simulink model "invers_dynamics_exo"  (R2023a)
settings: Solver=FixedStepAuto  StartTime=0.0  StopTime=20  RelTol=1e-3
libraries: simulink x6
settings Model: Creator=tobia  LastModifiedBy=tobia
settings OptimizationCC: OptimizeBlockIOStorage=off  ZeroExternalMemoryAtStartup=off  ZeroInternalMemoryAtStartup=off  OptimizeDataStoreBuffers=off  BusAssignmentInplaceUpdate=off
settings DebuggingCC: SFUnexpectedBacktrackingDiag=warning  SFNoUnconditionalDefaultTransitionDiag=warning
settings RTWCC: GenCodeOnly=on  GenerateReport=on  Toolchain=Microsoft Visual C++ 2022 v17.0 | CMake/nmake (64-bit Windows)  BuildConfiguration=Debug  LaunchReport=on  TargetLang=C++
settings CodeAppCC: ForceParamTrailComments=on  MATLABSourceComments=on  EnableCustomComments=on
settings GRTTargetCC: TargetLangStandard=C++11 (ISO)  CombineSignalStateStructs=on  CodeInterfacePackaging=C++ class  SupportVariableSizeSignals=on  MultiInstanceErrorCode=Warning

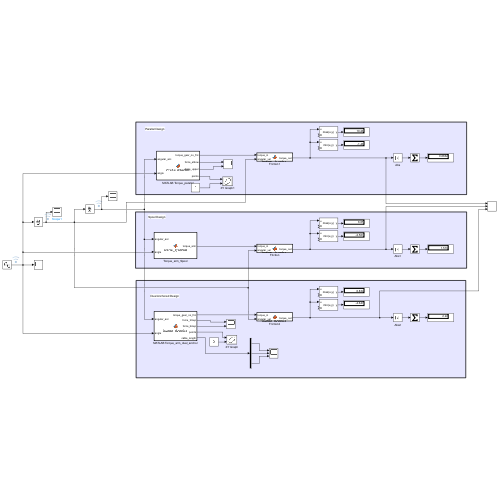
[thumbnail: Simulink's stored preview of the top-level diagram]
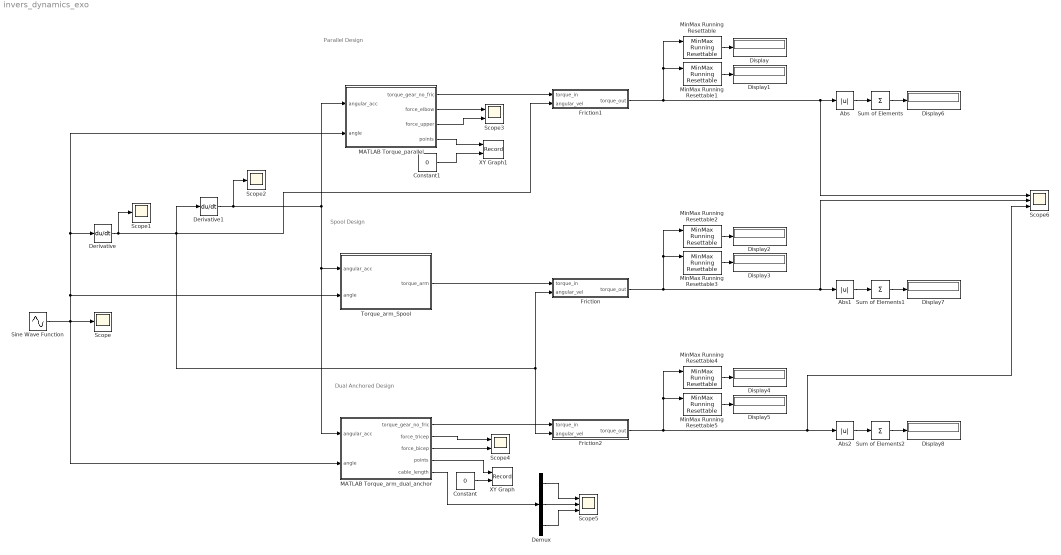
== system invers_dynamics_exo ==
  note: Dual Anchored Design
  note: Spool Design
  note: Parallel Design
  Abs : Abs  SaturateOnIntegerOverflow=off
  Abs1 : Abs  SaturateOnIntegerOverflow=off
  Abs2 : Abs  SaturateOnIntegerOverflow=off
  Constant : Constant  Value=0
  Constant1 : Constant  Value=0
  Demux : Demux  Outputs=3
  Derivative : Derivative
  Derivative1 : Derivative
  Display{,1..8} (9 alike) : Display
  Friction : MATLAB Function  TreatAsAtomicUnit=on
  Friction1 : MATLAB Function  TreatAsAtomicUnit=on
  Friction2 : MATLAB Function  TreatAsAtomicUnit=on
  MATLAB Torque_arm_dual_anchor : MATLAB Function  TreatAsAtomicUnit=on
  MATLAB Torque_parallel : MATLAB Function  TreatAsAtomicUnit=on
  MinMax Running Resettable : simulink/Math Operations/MinMax Running Resettable  Function=max  vinit=0.0
  MinMax Running Resettable1 : simulink/Math Operations/MinMax Running Resettable  Function=min  vinit=0.0
  MinMax Running Resettable2 : simulink/Math Operations/MinMax Running Resettable  Function=max  vinit=0.0
  MinMax Running Resettable3 : simulink/Math Operations/MinMax Running Resettable  Function=min  vinit=0.0
  MinMax Running Resettable4 : simulink/Math Operations/MinMax Running Resettable  Function=max  vinit=0.0
  MinMax Running Resettable5 : simulink/Math Operations/MinMax Running Resettable  Function=min  vinit=0.0
  Scope : Scope
  Scope1 : Scope
  Scope2 : Scope
  Scope3 : Scope  NumInputPorts=2
  Scope4 : Scope  NumInputPorts=2
  Scope5 : Scope  NumInputPorts=3
  Scope6 : Scope  NumInputPorts=3
  Sine Wave Function : Sin  Amplitude=57.5*pi/180  Bias=57.5*pi/180  Frequency=0.5  Phase=4  SampleTime=0.01
  Sum of Elements : Sum  Inputs=+
  Sum of Elements1 : Sum  Inputs=+
  Sum of Elements2 : Sum  Inputs=+
  Torque_arm_Spool : MATLAB Function  TreatAsAtomicUnit=on
  XY Graph : Record  FileSettingsInternal="{\"entries\":[{\"content\":{\"excelSettings\":{\"content\":{},\"type\":\"Streamout.ExcelSettings\"}},\"type\":\"Streamout.FileSettingStorage\",\"uuid\":\"90cafc74-587b-4871-8b77-8289e6956aa1\"}],\"packageUris\":[\"http://schema.mathworks.com/mf0/streamout_blocks/R2020a\"],\"version\":\"1.0\"}"  Layout=[1 1]  SignalsInternal="{\"entries\":[{\"content\":{\"signals\":[{\"content\":{\"blockPath\":[\"invers_dynamics_exo/XY Graph\"],\"dimensions\":[1,8],\"domain\":\"invers_dynamics_exo/XY Graph\",\"hasChildren\":true,\"lineColor\":\"#ff13a6\",\"port\":1,\"sid\":[\"\"],\"signalID\":426,\"signalName\":\"MATLAB Torque_arm_dual_anchor:4\"},\"type\":\"RecordBlkView.Signal\",\"uuid\":\"f57bbfb4-fc0c-47c9-ab87-1a3b218e2124\"},{\"content\":{\"blockPath\":[\"invers_dynamics_exo/XY Graph\"],\"channel\":[1,1],\"dimensions\":[1,8],\"domain\":\"invers_dynamics_exo/XY Graph\",\"lineColor\":\"#7e2f8e\",\"parentID\":426,\"plots\":[1],\"port\":1,\"sid\":[\"\"],\"signalID\":427,\"signalName\":\"MATLAB Torque_arm_dual_anchor:4\"},\"type\":\"RecordBlkView.Signal\",\"uuid\":\"17954e79-1570-4b7c-beb2-87390e5cb58c\"},{\"content\":{\"blockPath\":[\"invers_dynamics_exo/XY Graph\"],\"dimensions\":[1],\"domain\":\"invers_dynamics_exo/XY Graph\",\"lineColor\":\"#a2142f\",\"plots\":[1],\"port\":2,\"sid\":[\"\"],\"signalID\":436,\"signalName\":\"Constant\"},\"type\":\"RecordBlkView.Signal\",\"uuid\":\"88e606e6-8988-44ae-93fd-16471fbb4abb\"},{\"content\":{\"blockPath\":[\"invers_dynamics_exo/XY Graph\"],\"channel\":[1,2],\"dimensions\":[1,8],\"domain\":\"invers_dynamics_exo/XY Graph\",\"lineColor\":\"#64d413\",\"parentID\":426,\"plots\":[1],\"port\":1,\"sid\":[\"\"],\"signalID\":497,\"signalName\":\"MATLAB Torque_arm_dual_anchor:4\"},\"type\":\"RecordBlkView.Signal\",\"uuid\":\"809d9a61-5690-47a9-8092-efb78bb0c7b6\"},{\"content\":{\"blockPath\":[\"invers_dynamics_exo/XY Graph\"],\"channel\":[1,3],\"dimensions\":[1,8],\"domain\":\"invers_dynamics_exo/XY Graph\",\"lineColor\":\"#ff13a6\",\"parentID\":426,\"plots\":[1],\"port\":1,\"sid\":[\"\"],\"signalID\":498,\"signalName\":\"MATLAB Torque_arm_dual_anchor:4\"},\"type\":\"RecordBlkView.Signal\",\"uuid\":\"46f14f9b-1d62-4e7a-9e42-de28faff6f15\"},{\"content\":{\"blockPath\":[\"invers_dynamics_exo/XY Graph\"],\"channel\":[1,4],\"dimensions\":[1,8],\"domain\":\"invers_dynamics_exo/XY Graph\",\"lineColor\":\"#fe330a\",\"parentID\":426,\"plots\":[1],\"port\":1,\"sid\":[\"\"],\"signalID\":499,\"signalName\":\"MATLAB Torque_arm_dual_anchor:4\"},\"type\":\"RecordBlkView.Signal\",\"uuid\":\"354214a8-296c-4194-9ecc-28dd992aaaef\"},{\"content\":{\"blockPath\":[\"invers_dynamics_exo/XY Graph\"],\"channel\":[1,5],\"dimensions\":[1,8],\"domain\":\"invers_dynamics_exo/XY Graph\",\"lineColor\":\"#22b573\",\"parentID\":426,\"plots\":[1],\"port\":1,\"sid\":[\"\"],\"signalID\":500,\"signalName\":\"MATLAB Torque_arm_dual_anchor:4\"},\"type\":\"RecordBlkView.Signal\",\"uuid\":\"e2127789-c763-4787-91a7-13d7228fb6b6\"},{\"content\":{\"blockPath\":[\"invers_dynamics_exo/XY Graph\"],\"channel\":[1,6],\"dimensions\":[1,8],\"domain\":\"invers_dynamics_exo/XY Graph\",\"lineColor\":\"#0072bd\",\"parentID\":426,\"plots\":[1],\"port\":1,\"sid\":[\"\"],\"signalID\":501,\"signalName\":\"MATLAB Torque_arm_dual_anchor:4\"},\"type\":\"RecordBlkView.Signal\",\"uuid\":\"b365466d-55b6-410a-a4a0-64c454fc3450\"},{\"content\":{\"blockPath\":[\"invers_dynamics_exo/XY Graph\"],\"channel\":[1,7],\"dimensions\":[1,8],\"domain\":\"invers_dynamics_exo/XY Graph\",\"lineColor\":\"#d95319\",\"parentID\":426,\"plots\":[1],\"port\":1,\"sid\":[\"\"],\"signalID\":502,\"signalName\":\"MATLAB Torque_arm_dual_anchor:4\"},\"type\":\"RecordBlkView.Signal\",\"uuid\":\"c2ca46fb-f305-425c-9fde-4563dfa5b76e\"},{\"content\":{\"blockPath\":[\"invers_dynamics_exo/XY Graph\"],\"channel\":[1,8],\"dimensions\":[1,8],\"domain\":\"invers_dynamics_exo/XY Graph\",\"lineColor\":\"#edb120\",\"parentID\":426,\"plots\":[1],\"port\":1,\"sid\":[\"\"],\"signalID\":503,\"signalName\":\"MATLAB Torque_arm_dual_anchor:4\"},\"type\":\"RecordBlkView.Signal\",\"uuid\":\"76ece406-2e19-4193-9589-b77808bf0ec4\"}]},\"type\":\"RecordBlkView.InputSignals\",\"uuid\":\"c80cf8b0-44b7-4c38-9eaf-bf62f72da6b7\"}],\"packageUris\":[\"http://schema.mathworks.com/mf0/streamout_blocks/R2020a\"],\"version\":\"1.0\"}"  VisualizationBindings="{\"xyplotplugin\":{\"info\":[{\"series\":[{\"bindingParametersList\":[{\"parameter\":\"X-Axis\",\"signalID\":498,\"signalName\":\"MATLAB Torque_arm_dual_anchor:4(1,3)\"},{\"parameter\":\"Y-Axis\",\"signalID\":499,\"signalName\":\"MATLAB Torque_arm_dual_anchor:4(1,4)\"}],\"seriesID\":23966},{\"bindingParametersList\":[{\"parameter\":\"X-Axis\",\"signalID\":436,\"signalName\":\"Constant\"},{\"parameter\":\"Y-Axis\",\"signalID\":436,\"signalName\":\"Constant\"}],\"seriesID\":54397},{\"bindingParametersList\":[{\"parameter\":\"X-Axis\",\"signalID\":427,\"signalName\":\"MATLAB Torque_arm_dual_anchor:4(1,1)\"},{\"parameter\":\"Y-Axis\",\"signalID\":497,\"signalName\":\"MATLAB Torque_arm_dual_anchor:4(1,2)\"}],\"seriesID\":41728},{\"bindingParametersList\":[{\"parameter\":\"X-Axis\",\"signalID\":500,\"signalName\":\"MATLAB Torque_arm_dual_anchor:4(1,5)\"},{\"parameter\":\"Y-Axis\",\"signalID\":501,\"signalName\":\"MATLAB Torque_arm_dual_anchor:4(1,6)\"}],\"seriesID\":13745},{\"bindingParametersList\":[{\"parameter\":\"X-Axis\",\"signalID\":502,\"signalName\":\"MATLAB Torque_arm_dual_anchor:4(1,7)\"},{\"parameter\":\"Y-Axis\",\"signalID\":503,\"signalName\":\"MATLAB Torque_arm_dual_anchor:4(1,8)\"}],\"seriesID\":51218}],\"subplotID\":1}]}}"  CompatibilityTag=XY
  XY Graph1 : Record  FileSettingsInternal="{\"entries\":[{\"content\":{\"excelSettings\":{\"content\":{},\"type\":\"Streamout.ExcelSettings\"}},\"type\":\"Streamout.FileSettingStorage\",\"uuid\":\"f9a8d002-46d0-471b-8204-3856352c4768\"}],\"packageUris\":[\"http://schema.mathworks.com/mf0/streamout_blocks/R2020a\"],\"version\":\"1.0\"}"  Layout=[1 1]  SignalsInternal="{\"entries\":[{\"content\":{\"signals\":[{\"content\":{\"blockPath\":[\"invers_dynamics_exo/XY Graph1\"],\"dimensions\":[1,8],\"domain\":\"invers_dynamics_exo/XY Graph1\",\"hasChildren\":true,\"lineColor\":\"#22b573\",\"port\":1,\"sid\":[\"\"],\"signalID\":431,\"signalName\":\"MATLAB Torque_parallel:4\"},\"type\":\"RecordBlkView.Signal\",\"uuid\":\"b3d6e127-3aca-4ccc-b929-aedfbef8128b\"},{\"content\":{\"blockPath\":[\"invers_dynamics_exo/XY Graph1\"],\"channel\":[1,1],\"dimensions\":[1,8],\"domain\":\"invers_dynamics_exo/XY Graph1\",\"lineColor\":\"#4dbeee\",\"parentID\":431,\"plots\":[1],\"port\":1,\"sid\":[\"\"],\"signalID\":432,\"signalName\":\"MATLAB Torque_parallel:4\"},\"type\":\"RecordBlkView.Signal\",\"uuid\":\"55e012bc-9410-4221-816c-c6f02a738b49\"},{\"content\":{\"blockPath\":[\"invers_dynamics_exo/XY Graph1\"],\"dimensions\":[1],\"domain\":\"invers_dynamics_exo/XY Graph1\",\"lineColor\":\"#139fff\",\"plots\":[1],\"port\":2,\"sid\":[\"\"],\"signalID\":440,\"signalName\":\"Constant1\"},\"type\":\"RecordBlkView.Signal\",\"uuid\":\"e45e3ae8-e52d-4690-83d0-35f4cc038db9\"},{\"content\":{\"blockPath\":[\"invers_dynamics_exo/XY Graph1\"],\"channel\":[1,2],\"dimensions\":[1,8],\"domain\":\"invers_dynamics_exo/XY Graph1\",\"lineColor\":\"#7e2f8e\",\"parentID\":431,\"plots\":[1],\"port\":1,\"sid\":[\"\"],\"signalID\":465,\"signalName\":\"MATLAB Torque_parallel:4\"},\"type\":\"RecordBlkView.Signal\",\"uuid\":\"faa6bfa9-b2c7-49a6-80bf-c0cf82e5d0fc\"},{\"content\":{\"blockPath\":[\"invers_dynamics_exo/XY Graph1\"],\"channel\":[1,3],\"dimensions\":[1,8],\"domain\":\"invers_dynamics_exo/XY Graph1\",\"lineColor\":\"#77ac30\",\"parentID\":431,\"plots\":[1],\"port\":1,\"sid\":[\"\"],\"signalID\":466,\"signalName\":\"MATLAB Torque_parallel:4\"},\"type\":\"RecordBlkView.Signal\",\"uuid\":\"3d7e6bb0-1d54-4c15-bab5-21ddea2239ad\"},{\"content\":{\"blockPath\":[\"invers_dynamics_exo/XY Graph1\"],\"channel\":[1,4],\"dimensions\":[1,8],\"domain\":\"invers_dynamics_exo/XY Graph1\",\"lineColor\":\"#4dbeee\",\"parentID\":431,\"plots\":[1],\"port\":1,\"sid\":[\"\"],\"signalID\":467,\"signalName\":\"MATLAB Torque_parallel:4\"},\"type\":\"RecordBlkView.Signal\",\"uuid\":\"c57de7f5-fb7a-4800-a95d-2f3c6294c59a\"},{\"content\":{\"blockPath\":[\"invers_dynamics_exo/XY Graph1\"],\"channel\":[1,5],\"dimensions\":[1,8],\"domain\":\"invers_dynamics_exo/XY Graph1\",\"lineColor\":\"#a2142f\",\"parentID\":431,\"plots\":[1],\"port\":1,\"sid\":[\"\"],\"signalID\":468,\"signalName\":\"MATLAB Torque_parallel:4\"},\"type\":\"RecordBlkView.Signal\",\"uuid\":\"42b639ed-fed3-4663-bc29-7e429b7bdf60\"},{\"content\":{\"blockPath\":[\"invers_dynamics_exo/XY Graph1\"],\"channel\":[1,6],\"dimensions\":[1,8],\"domain\":\"invers_dynamics_exo/XY Graph1\",\"lineColor\":\"#139fff\",\"parentID\":431,\"plots\":[1],\"port\":1,\"sid\":[\"\"],\"signalID\":469,\"signalName\":\"MATLAB Torque_parallel:4\"},\"type\":\"RecordBlkView.Signal\",\"uuid\":\"2b51fe8f-0079-4332-86c0-0fcd8a819aaa\"},{\"content\":{\"blockPath\":[\"invers_dynamics_exo/XY Graph1\"],\"channel\":[1,7],\"dimensions\":[1,8],\"domain\":\"invers_dynamics_exo/XY Graph1\",\"lineColor\":\"#ff6929\",\"parentID\":431,\"plots\":[1],\"port\":1,\"sid\":[\"\"],\"signalID\":470,\"signalName\":\"MATLAB Torque_parallel:4\"},\"type\":\"RecordBlkView.Signal\",\"uuid\":\"4737f375-8d5a-41d0-90f0-dd112fd7b9d5\"},{\"content\":{\"blockPath\":[\"invers_dynamics_exo/XY Graph1\"],\"channel\":[1,8],\"dimensions\":[1,8],\"domain\":\"invers_dynamics_exo/XY Graph1\",\"lineColor\":\"#b746ff\",\"parentID\":431,\"plots\":[1],\"port\":1,\"sid\":[\"\"],\"signalID\":471,\"signalName\":\"MATLAB Torque_parallel:4\"},\"type\":\"RecordBlkView.Signal\",\"uuid\":\"66e42e63-d3ff-4148-a1e3-97cb48d4e207\"}]},\"type\":\"RecordBlkView.InputSignals\",\"uuid\":\"e7de4f62-20f8-44cb-8264-9c3d469c1695\"}],\"packageUris\":[\"http://schema.mathworks.com/mf0/streamout_blocks/R2020a\"],\"version\":\"1.0\"}"  VisualizationBindings="{\"xyplotplugin\":{\"info\":[{\"series\":[{\"bindingParametersList\":[{\"parameter\":\"X-Axis\",\"signalID\":470,\"signalName\":\"MATLAB Torque_parallel:4(1,7)\"},{\"parameter\":\"Y-Axis\",\"signalID\":471,\"signalName\":\"MATLAB Torque_parallel:4(1,8)\"}],\"seriesID\":52874},{\"bindingParametersList\":[{\"parameter\":\"X-Axis\",\"signalID\":466,\"signalName\":\"MATLAB Torque_parallel:4(1,3)\"},{\"parameter\":\"Y-Axis\",\"signalID\":467,\"signalName\":\"MATLAB Torque_parallel:4(1,4)\"}],\"seriesID\":24947},{\"bindingParametersList\":[{\"parameter\":\"X-Axis\",\"signalID\":432,\"signalName\":\"MATLAB Torque_parallel:4(1,1)\"},{\"parameter\":\"Y-Axis\",\"signalID\":465,\"signalName\":\"MATLAB Torque_parallel:4(1,2)\"}],\"seriesID\":9866},{\"bindingParametersList\":[{\"parameter\":\"X-Axis\",\"signalID\":468,\"signalName\":\"MATLAB Torque_parallel:4(1,5)\"},{\"parameter\":\"Y-Axis\",\"signalID\":469,\"signalName\":\"MATLAB Torque_parallel:4(1,6)\"}],\"seriesID\":40053}],\"subplotID\":1}]}}"  CompatibilityTag=XY
  wires:
  Sine Wave Function/1 -> MATLAB Torque_parallel/2(angle), Derivative/1, Torque_arm_Spool/2(angle), Scope/1, MATLAB Torque_arm_dual_anchor/2(angle)
  Derivative/1 -> Scope1/1, Friction2/2(angular_vel), Friction/2(angular_vel), Friction1/2(angular_vel), Derivative1/1
  Derivative1/1 -> Scope2/1, MATLAB Torque_arm_dual_anchor/1(angular_acc), Torque_arm_Spool/1(angular_acc), MATLAB Torque_parallel/1(angular_acc)
  MATLAB Torque_parallel/1(torque_gear_no_fric) -> Friction1/1(torque_in)
  MATLAB Torque_parallel/4(points) -> XY Graph1/1
  Torque_arm_Spool/1(torque_arm) -> Friction/1(torque_in)
  Constant1/1 -> XY Graph1/2
  MATLAB Torque_arm_dual_anchor/4(points) -> XY Graph/1
  MATLAB Torque_arm_dual_anchor/1(torque_gear_no_fric) -> Friction2/1(torque_in)
  MATLAB Torque_arm_dual_anchor/5(cable_length) -> Demux/1
  Constant/1 -> XY Graph/2
  MATLAB Torque_parallel/3(force_upper) -> Scope3/2
  MATLAB Torque_parallel/2(force_elbow) -> Scope3/1
  MATLAB Torque_arm_dual_anchor/3(force_bicep) -> Scope4/2
  MATLAB Torque_arm_dual_anchor/2(force_tricep) -> Scope4/1
  Demux/1 -> Scope5/1
  Demux/2 -> Scope5/2
  Demux/3 -> Scope5/3
  Friction1/1(torque_out) -> MinMax Running Resettable1/1, MinMax Running Resettable/1, Abs/1, Scope6/1
  MinMax Running Resettable/1 -> Display/1
  MinMax Running Resettable1/1 -> Display1/1
  MinMax Running Resettable3/1 -> Display3/1
  MinMax Running Resettable2/1 -> Display2/1
  MinMax Running Resettable5/1 -> Display5/1
  MinMax Running Resettable4/1 -> Display4/1
  Abs/1 -> Sum of Elements/1
  Abs1/1 -> Sum of Elements1/1
  Friction/1(torque_out) -> Scope6/2, Abs1/1, MinMax Running Resettable3/1, MinMax Running Resettable2/1
  Abs2/1 -> Sum of Elements2/1
  Friction2/1(torque_out) -> Abs2/1, Scope6/3, MinMax Running Resettable5/1, MinMax Running Resettable4/1
  Sum of Elements/1 -> Display6/1
  Sum of Elements2/1 -> Display8/1
  Sum of Elements1/1 -> Display7/1

== matlab function invers_dynamics_exo/MATLAB Torque_arm_dual_anchor ==
  data: angular_acc input; torque_gear_no_fric output; angle input; force_tricep output; force_bicep output; points output; cable_length output
function [torque_gear_no_fric, force_tricep, force_bicep, points, cable_length]= inverse_dynamics(angular_acc, angle)
% arm data
mass_arm = 1.134; % kg
exo_mass = 0.05457; % kg
total_mass_arm = mass_arm + exo_mass;

length_arm = 0.3; % m
cylinder_radius = 0.025; % m

% other
g = 9.82; 
mass_end_effector = 1; % kg

I = (total_mass_arm * length_arm^2) / 3;

tynde_moment = -((length_arm/2) * total_mass_arm * g * cos(angle));

payload_moment = -(length_arm * mass_end_effector * g * cos(angle));

torque_arm = I * angular_acc - tynde_moment - payload_moment;
% torque_arm = I * angular_acc;

%% Static anchorpoints
Anchorpoint_uperarm_bicep = [-0.03375, 0.02145];
Anchorpoint_uperarm_tricep = [0.03533,-0.05673]; 

%% Max exstention of the lower arm piece's anchorpoints 

rotation_z = [cos(angle), sin(angle); -sin(angle), cos(angle)];
Anchorpoint_lowerarm_bicep = [0.12893,0.03573]*rotation_z;
Anchorpoint_lowerarm_tricep =[0.136,-0.030]*rotation_z;

%% Making the two vectors between pair of anchorpoints
bicep_vector =  Anchorpoint_lowerarm_bicep-Anchorpoint_uperarm_bicep   ;
tricep_vector =  Anchorpoint_lowerarm_tricep- Anchorpoint_uperarm_tricep ;

bicep_cable_length = norm(bicep_vector) - 0.1441;
tricep_cable_length = norm(tricep_vector) - 0.1441;
cable_length_diff = abs(tricep_cable_length+bicep_cable_length);
cable_length = [bicep_cable_length, tricep_cable_length, cable_length_diff];

%%
bicep_vector_cross = norm(cross([Anchorpoint_lowerarm_bicep(1), Anchorpoint_lowerarm_bicep(2), 0],[bicep_vector(1), bicep_vector(2), 0]));
bicep_vector_dist_origin = bicep_vector_cross / (norm(bicep_vector));

%%
tricep_vector_cross = norm(cross([Anchorpoint_lowerarm_tricep(1), Anchorpoint_lowerarm_tricep(2), 0],[tricep_vector(1), tricep_vector(2), 0]));
tricep_vector_dist_origin = tricep_vector_cross / (norm(tricep_vector));

if torque_arm > 0
    force = torque_arm / bicep_vector_dist_origin;
else 
    force = torque_arm / tricep_vector_dist_origin;
end

torque_gear_no_fric = force * cylinder_radius;



if force > 0
    force_bicep = force;
    force_tricep = 0;
else
    force_tricep = -force;
    force_bicep = 0;
end

points = [Anchorpoint_uperarm_tricep,Anchorpoint_uperarm_bicep,Anchorpoint_lowerarm_tricep,Anchorpoint_lowerarm_bicep];

== matlab function invers_dynamics_exo/Torque_arm_Spool ==
  data: angular_acc input; torque_arm output; angle input
function torque_arm = inverse_dynamics(angular_acc, angle)
% arm data
mass_arm = 1.134; % kg
exo_mass = 0.05457; % kg
total_mass_arm = mass_arm + exo_mass;

length_arm = 0.3; % m
% cylinder_radius = 0.025; % m

% other
g = 9.82; 
mass_end_effector = 1; % kg

I = (total_mass_arm * length_arm^2) / 3;

tynde_moment = -((length_arm/2) * total_mass_arm * g * cos(angle))

payload_moment = -(length_arm * mass_end_effector * g * cos(angle));

torque_arm = I * angular_acc - tynde_moment - payload_moment;

== matlab function invers_dynamics_exo/Friction ==
  data: torque_in input; angular_vel input; torque_out output
function torque_out = inverse_dynamics(torque_in, angular_vel)
mu = 0.04;
phi = 2*pi;

torque_out = torque_in / exp(-mu*phi*sign(angular_vel)*sign(torque_in));

== matlab function invers_dynamics_exo/Friction2 ==
  data: torque_in input; angular_vel input; torque_out output
function torque_out = inverse_dynamics(torque_in, angular_vel)
mu = 0.04;
phi = 2*pi + pi/4 + pi/2;
%torque_arm = 1;
torque_out = torque_in / exp(-mu*phi*sign(angular_vel)*sign(torque_in));

== matlab function invers_dynamics_exo/MATLAB Torque_parallel ==
  data: angular_acc input; torque_gear_no_fric output; angle input; force_elbow output; force_upper output; points output
function [torque_gear_no_fric, force_elbow, force_upper, points]= inverse_dynamics(angular_acc, angle)
% arm data
mass_arm = 1.134; % kg
exo_mass = 0.05457; % kg
total_mass_arm = mass_arm + exo_mass;

length_arm = 0.3; % m
cylinder_radius = 0.025; % m

% other
g = 9.82; 
mass_end_effector = 1; % kg

I = (total_mass_arm * length_arm^2) / 3;

tau_gravity = -((length_arm/2) * total_mass_arm * g * cos(angle));

tau_payload = -(length_arm * mass_end_effector * g * cos(angle));

torque_arm = I * angular_acc - tau_gravity - tau_payload;
% torque_arm = I * angular_acc;

%% Static anchorpoints
Anchorpoint_upper = [-0.1154,0.0331];
Anchorpoint_elbow = [0,0]; 

%% Max exstention of the lower arm piece's anchorpoints 

rotation_z = [cos(angle), sin(angle); -sin(angle), cos(angle)];
Anchorpoint_lower = [0.12, 0.]*rotation_z;
Anchorpoint_free = Anchorpoint_lower+[-0.1154, 0.0331];

%% Making the two vectors between pair of anchorpoints
upper_vector =  Anchorpoint_lower-Anchorpoint_upper  ;
elbow_vector =  Anchorpoint_free- Anchorpoint_elbow ;

%%
elbow_vector_cross = norm(cross([Anchorpoint_lower(1), Anchorpoint_lower(2), 0],[upper_vector(1), upper_vector(2), 0]));
elbow_vector_dist_origin = elbow_vector_cross / (norm(upper_vector));

%%
upper_vector_cross = norm(cross(([-0.1154, 0.0331, 0]+[Anchorpoint_free(1), Anchorpoint_free(2), 0]),[elbow_vector(1), elbow_vector(2), 0]));
upper_vector_dist_origin = upper_vector_cross / (norm(elbow_vector));

if torque_arm > 0
    force = torque_arm / elbow_vector_dist_origin;
else 
    force = torque_arm / upper_vector_dist_origin;
end

torque_gear_no_fric = force * cylinder_radius;



if force > 0
    force_upper = force;
    force_elbow = 0;
else
    force_elbow = -force;
    force_upper = 0;
end

points = [Anchorpoint_elbow,Anchorpoint_upper,Anchorpoint_free,Anchorpoint_lower];

== matlab function invers_dynamics_exo/Friction1 ==
  data: torque_in input; angular_vel input; torque_out output
function torque_out = inverse_dynamics(torque_in, angular_vel)
mu = 0.04;
phi = pi + 2*pi;
%torque_arm = 1;
torque_out = torque_in / exp(-mu*phi*sign(angular_vel)*sign(torque_in));
